simulink model "navigator2"  (R2013b)
settings: Solver=ode45  StartTime=0.0  StopTime=inf  RelTol=1e-3
undefined symbols (not defined in the file): Earth, WGS84
libraries: aerolibtransform2 x4
settings Model: Creator=Gianluca Rossetti  LastModifiedBy=Gianluca Rossetti

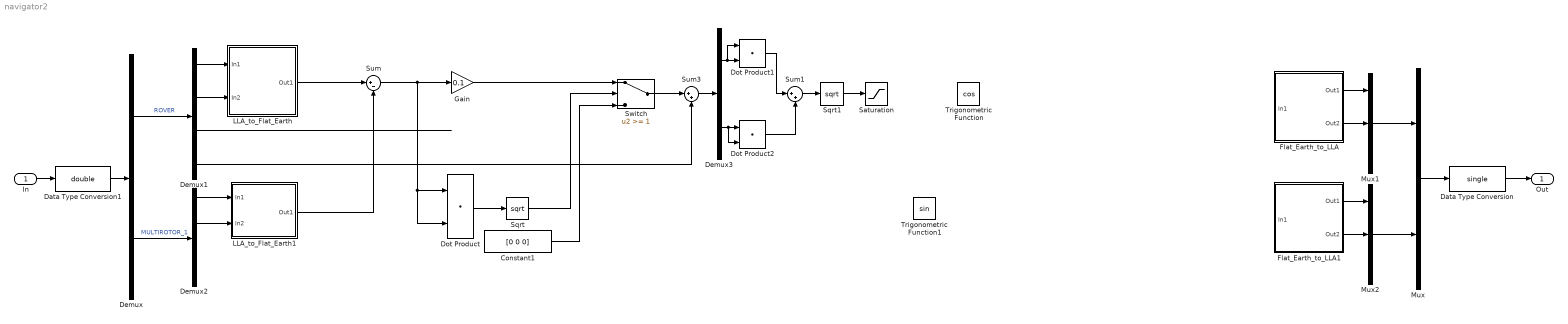
== system navigator2 ==
  In : Inport
  Constant1 : Constant  Value=[0 0 0]
  Data Type Conversion : DataTypeConversion  OutDataTypeStr=single
  Data Type Conversion1 : DataTypeConversion  OutDataTypeStr=double
  Demux : Demux  Outputs=[7 7]
  Demux1 : Demux  Outputs=[2 1 2 2]
  Demux2 : Demux  Outputs=[2 1 2 2]
  Demux3 : Demux  Outputs=[1 1]
  Dot Product : DotProduct  InputSameDT=on  OutDataTypeStr=Inherit: Inherit via internal rule
  Dot Product1 : DotProduct  InputSameDT=on  OutDataTypeStr=Inherit: Inherit via internal rule
  Dot Product2 : DotProduct  InputSameDT=on  OutDataTypeStr=Inherit: Inherit via internal rule
  Flat_Earth_to_LLA : Subsystem
  Flat_Earth_to_LLA1 : Subsystem
  Gain : Gain  Gain=0.1
  LLA_to_Flat_Earth : Subsystem
  LLA_to_Flat_Earth1 : Subsystem
  Mux : Mux  Inputs=[5 5]
  Mux1 : Mux  Inputs=[2 1 2]
  Mux2 : Mux  Inputs=[2 1 2]
  Saturation : Saturate  UpperLimit=10  LowerLimit=0
  Sqrt : Sqrt  SaturateOnIntegerOverflow=on
  Sqrt1 : Sqrt  SaturateOnIntegerOverflow=on
  Sum : Sum  Inputs=|+-
  Sum1 : Sum  Inputs=|++
  Sum3 : Sum  Inputs=|++
  Switch : Switch  Threshold=1
  Trigonometric Function : Trigonometry  Operator=cos
  Trigonometric Function1 : Trigonometry
  Out : Outport
  wires:
  Demux/1 -> Demux1/1  "ROVER"
  In/1 -> Data Type Conversion1/1
  Data Type Conversion1/1 -> Demux/1
  Mux1/1 -> Mux/1
  Demux1/1 -> LLA_to_Flat_Earth/1(In1)
  Demux1/2 -> LLA_to_Flat_Earth/2(In2)
  Flat_Earth_to_LLA/1(Out1) -> Mux1/1
  Flat_Earth_to_LLA/2(Out2) -> Mux1/2
  Data Type Conversion/1 -> Out/1
  Mux/1 -> Data Type Conversion/1
  Demux/2 -> Demux2/1  "MULTIROTOR_1"
  Mux2/1 -> Mux/2
  Demux2/1 -> LLA_to_Flat_Earth1/1(In1)
  Demux2/2 -> LLA_to_Flat_Earth1/2(In2)
  Flat_Earth_to_LLA1/1(Out1) -> Mux2/1
  Flat_Earth_to_LLA1/2(Out2) -> Mux2/2
  LLA_to_Flat_Earth/1(Out1) -> Sum/1
  LLA_to_Flat_Earth1/1(Out1) -> Sum/2
  Sum/1 -> Dot Product/2, Dot Product/1, Gain/1
  Demux1/4 -> Sum3/2
  Dot Product/1 -> Sqrt/1
  Sqrt/1 -> Switch/2
  Constant1/1 -> Switch/3
  Switch/1 -> Sum3/1
  Gain/1 -> Switch/1
  Sum3/1 -> Demux3/1
  Demux3/2 -> Dot Product2/2, Dot Product2/1
  Demux3/1 -> Dot Product1/1, Dot Product1/2
  Dot Product1/1 -> Sum1/1
  Dot Product2/1 -> Sum1/2
  Sum1/1 -> Sqrt1/1
  Sqrt1/1 -> Saturation/1
  Demux1/3 -> ?

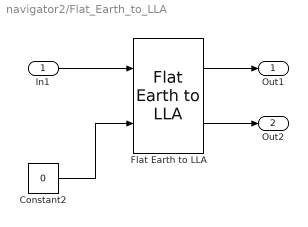
== system navigator2/Flat_Earth_to_LLA ==
  In1 : Inport
  Constant2 : Constant  Value=0  OutDataTypeStr=single
  Flat Earth to LLA : aerolibtransform2/Flat Earth to LLA  units=Metric (MKS)  ptype=Earth (WGS84)  F=1/298.257223563  R=6378137  LL0="[44.201892800000003  12.062565800000000]"  psi=0
  Out1 : Outport
  Out2 : Outport  Port=2
  wires:
  Flat Earth to LLA/1 -> Out1/1
  In1/1 -> Flat Earth to LLA/1
  Constant2/1 -> Flat Earth to LLA/2
  Flat Earth to LLA/2 -> Out2/1

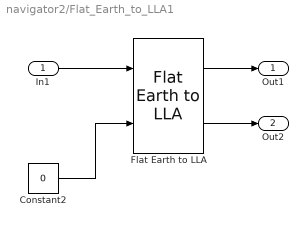
== system navigator2/Flat_Earth_to_LLA1 ==
  In1 : Inport
  Constant2 : Constant  Value=0  OutDataTypeStr=single
  Flat Earth to LLA : aerolibtransform2/Flat Earth to LLA  units=Metric (MKS)  ptype=Earth (WGS84)  F=1/298.257223563  R=6378137  LL0="[44.201892800000003  12.062565800000000]"  psi=0
  Out1 : Outport
  Out2 : Outport  Port=2
  wires:
  Flat Earth to LLA/2 -> Out2/1
  Constant2/1 -> Flat Earth to LLA/2
  In1/1 -> Flat Earth to LLA/1
  Flat Earth to LLA/1 -> Out1/1

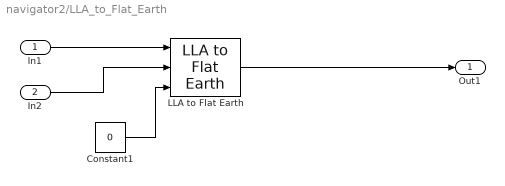
== system navigator2/LLA_to_Flat_Earth ==
  In1 : Inport
  In2 : Inport  Port=2
  Constant1 : Constant  Value=0  OutDataTypeStr=single
  LLA to Flat Earth : aerolibtransform2/LLA to Flat Earth  units=Metric (MKS)  ptype=Earth (WGS84)  F=1/298.257223563  R=6378137  LL0="[44.201892800000003  12.062565800000000]"  psi=0
  Out1 : Outport
  wires:
  In1/1 -> LLA to Flat Earth/1
  In2/1 -> LLA to Flat Earth/2
  Constant1/1 -> LLA to Flat Earth/3
  LLA to Flat Earth/1 -> Out1/1

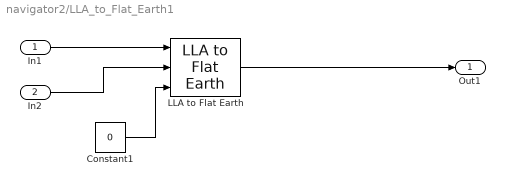
== system navigator2/LLA_to_Flat_Earth1 ==
  In1 : Inport
  In2 : Inport  Port=2
  Constant1 : Constant  Value=0  OutDataTypeStr=single
  LLA to Flat Earth : aerolibtransform2/LLA to Flat Earth  units=Metric (MKS)  ptype=Earth (WGS84)  F=1/298.257223563  R=6378137  LL0="[44.201892800000003  12.062565800000000]"  psi=0
  Out1 : Outport
  wires:
  LLA to Flat Earth/1 -> Out1/1
  Constant1/1 -> LLA to Flat Earth/3
  In2/1 -> LLA to Flat Earth/2
  In1/1 -> LLA to Flat Earth/1
